simulink model "L7E1b"  (R2020b)
settings: Solver=VariableStepAuto  StartTime=0.0  StopTime=0.04  MaxStep=1e-6  RelTol=1e-3
libraries: powerlib x9
settings Model: Creator=Vedant Nath  LastModifiedBy=Vedant Nath
settings DataIOCC: ReturnWorkspaceOutputs=off

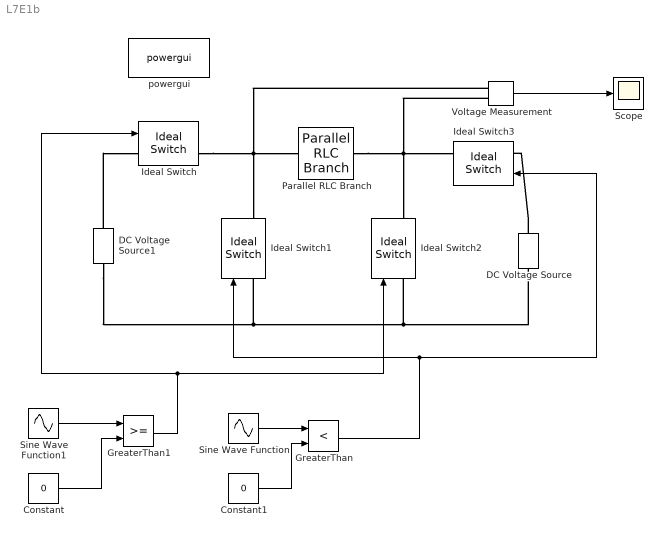
== system L7E1b ==
  Constant : Constant  Value=0
  Constant1 : Constant  Value=0
  DC Voltage Source : powerlib/Electrical Sources/DC Voltage Source  Amplitude=100  Measurements=None
  DC Voltage Source1 : powerlib/Electrical Sources/DC Voltage Source  Amplitude=100  Measurements=None
  GreaterThan : RelationalOperator  Operator=<  OutDataTypeStr=boolean  RndMeth=Simplest
  GreaterThan1 : RelationalOperator  OutDataTypeStr=boolean  RndMeth=Simplest
  Ideal Switch{,1..3} (4 alike) : powerlib/Power Electronics/Ideal Switch  Ron=0.001  Lon=0  IC=0  Rs=1e5  Cs=inf  Measurements=on
  Parallel RLC Branch : powerlib/Elements/Parallel RLC Branch  LConnTagsString=a  RConnTagsString=__new0  BranchType=R  Resistance=10  Inductance=1e-3  SetiL0=off  InitialCurrent=0  Capacitance=1e-6  Setx0=off  InitialVoltage=0  Measurements=None
  Scope : Scope
  Sine Wave Function : Sin  Frequency=314  SampleTime=0
  Sine Wave Function1 : Sin  Frequency=314  SampleTime=0
  Voltage Measurement : powerlib/Measurements/Voltage Measurement  PhasorSimulation=off  OutputType=Complex  PSBequivalent=0
  powergui : powerlib/powergui  Priority=1  SimulationMode=Continuous  SampleTime=50e-6  frequency=60  Iterations=50  frequencyindice=0  Pbase=100e6  ErrMax=1e-4  UnitsV=kV  UnitsW=MW  buscounter=0  FunctionMessages=off  echomessages=off  EnableUseOfTLC=off  CurrentSourceSwitches=off  DisableSnubberDevices=off  DisableRonSwitches=off  DisableVfSwitches=off  DisplayEquations=off  AutomaticDiscreteSolvers=off  SolverType=Tustin/Backward Euler (TBE)  Interpol=off  ExternalGateDelay=off  methode=off  Ts=100  x0status=zero  SPID=on  SwTol=0  HookPort=off  NonlinearTolerance=1e-4  nMaxIteration=100  ContinueOnMaxIteration=off  RestoreLinks=warning  ResistiveCurrentMeasurement=off  Frange=[0:2:500]  Ylog=off  Xlog=on  ShowGrid=off  save=off  variable=ZData  structure=ScopeData  ZoomFFT=off  StartTime=0.08  cycles=6  DisplayStyle=1  fundamental=50  FreqAxis=off  MaxFrequency=1500  frequencyindicesteady=1  RmsSteady=1  display=off
  wires:
  GreaterThan/1 -> Ideal Switch1/1, Ideal Switch3/1
  GreaterThan1/1 -> Ideal Switch/1, Ideal Switch2/1
  Voltage Measurement/1 -> Scope/1
  Sine Wave Function/1 -> GreaterThan/1
  Sine Wave Function1/1 -> GreaterThan1/1
  Constant/1 -> GreaterThan1/2
  Constant1/1 -> GreaterThan/2
  connections:
  Ideal Switch/RConn1 -- Parallel RLC Branch/LConn1 -- Voltage Measurement/LConn1 -- Ideal Switch1/RConn1
  Parallel RLC Branch/RConn1 -- Ideal Switch3/RConn1 -- Voltage Measurement/LConn2 -- Ideal Switch2/RConn1
  DC Voltage Source1/RConn1 -- Ideal Switch/LConn1
  DC Voltage Source/RConn1 -- Ideal Switch3/LConn1
  DC Voltage Source1/LConn1 -- Ideal Switch1/LConn1 -- Ideal Switch2/LConn1 -- DC Voltage Source/LConn1
